simulink model "export_archive_exec"  (Simulink 3.00)
libraries: execlib x5

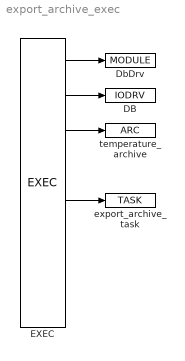
== system export_archive_exec ==
  DB : execlib/IODRV  module=DbDrv  classname=DbDrv  cfgname=export_archive.rio  factor=200  stack=10240  pri=3  timer=off
  DbDrv : execlib/MODULE
  EXEC : execlib/EXEC  target=PC - Linux  tick=0.05  ntick0=2  ntick1=50  ntick2=100  ntick3=1200  pri0=5  pri1=9  pri2=13  pri3=18
  export_archive_task : execlib/TASK  factor=1  start=0  stop=1  stack=10240  MDLOPEN=on
  temperature_archive : execlib/ARC  atype=1: RAM memory  asize=102400  nmarks=720  ldaymax=1048576  period=60
  wires:
  EXEC/1 -> DbDrv/1
  EXEC/2 -> DB/1
  EXEC/3 -> temperature_archive/1
  EXEC/5 -> export_archive_task/1
